simulink model "mobilesim1model"  (Simulink 6.6)
settings: Solver=ode3  StartTime=0.0  StopTime=100  FixedStep=dt  RelTol=1e-3
values from neighbouring files (symbols this model uses):
  D = 0.5    [mobile10demo.m]    (also in mobile2demo.m; mobilesim1demo.m; traje4demo.m = 1; vehi1demo.m)
  dt = 0.1    [mobile10demo.m]    (also in mobile2demo.m = 1; mobilesim1demo.m; traje1demo.m; traje2demo.m)
  theta0 = x0    [mobilesim1demo.m]
  xy = [x0(:),y0(:)]    [mobilesim1demo.m]
libraries: simulink x2
settings Model: Creator=root  LastModifiedBy=root
settings DebuggingCC: SignalResolutionControl=TryResolveAllWithWarning  MultiTaskDSMMsg=warning  MultiTaskCondExecSysMsg=none
settings RTWCC: IncludeERTFirstTime=on

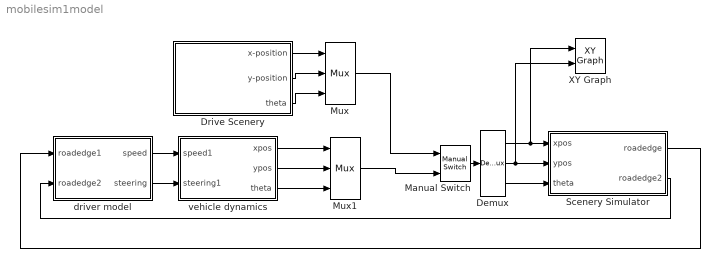
== system mobilesim1model ==
  Demux : Demux  Outputs=3
  Drive Scenery : Subsystem
  Manual Switch : simulink/Signal Routing/Manual Switch  SystemSampleTime=-1  sw=0  action=0  varsize=off
  Mux : Mux  Inputs=3
  Mux1 : Mux  Inputs=3
  Scenery Simulator : Subsystem
  XY Graph : simulink/Sinks/XY Graph  SystemSampleTime=-1  xmin=0  xmax=100  ymin=0  ymax=100  st=-1
  driver model : Subsystem
  vehicle dynamics : Subsystem
  wires:
  driver model/2(steering) -> vehicle dynamics/2(steering1)
  Scenery Simulator/2(roadedge2) -> driver model/2(roadedge2)
  Scenery Simulator/1(roadedge) -> driver model/1(roadedge1)
  driver model/1(speed) -> vehicle dynamics/1(speed1)
  Demux/1 -> Scenery Simulator/1(xpos), XY Graph/1
  Demux/2 -> Scenery Simulator/2(ypos), XY Graph/2
  Demux/3 -> Scenery Simulator/3(theta)
  Manual Switch/1 -> Demux/1
  vehicle dynamics/1(xpos) -> Mux1/1
  vehicle dynamics/2(ypos) -> Mux1/2
  vehicle dynamics/3(theta) -> Mux1/3
  Mux1/1 -> Manual Switch/2
  Mux/1 -> Manual Switch/1
  Drive Scenery/3(theta) -> Mux/3
  Drive Scenery/2(y-position) -> Mux/2
  Drive Scenery/1(x-position) -> Mux/1

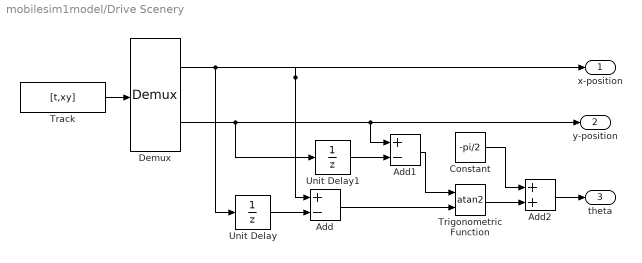
== system mobilesim1model/Drive Scenery ==
  Add : Sum  Inputs=+-  OutScaling=2^-10
  Add1 : Sum  Inputs=+-  OutScaling=2^-10
  Add2 : Sum  OutScaling=2^-10
  Constant : Constant  Value=-pi/2
  Demux : Demux  Outputs=2
  Track : FromWorkspace  VariableName=[t,xy]  SampleTime=dt
  Trigonometric Function : Trigonometry  Operator=atan2
  Unit Delay : UnitDelay  SampleTime=-1
  Unit Delay1 : UnitDelay  SampleTime=-1
  x-position : Outport
  y-position : Outport  Port=2
  theta : Outport  Port=3
  wires:
  Demux/2 -> Unit Delay1/1, y-position/1, Add1/1
  Demux/1 -> Unit Delay/1, Add/1, x-position/1
  Track/1 -> Demux/1
  Unit Delay/1 -> Add/2
  Add2/1 -> theta/1
  Constant/1 -> Add2/1
  Trigonometric Function/1 -> Add2/2
  Add/1 -> Trigonometric Function/2
  Add1/1 -> Trigonometric Function/1
  Unit Delay1/1 -> Add1/2

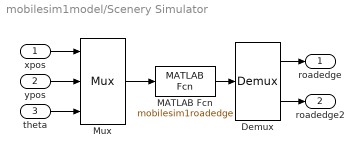
== system mobilesim1model/Scenery Simulator ==
  xpos : Inport
  ypos : Inport  Port=2
  theta : Inport  Port=3
  Demux : Demux  Outputs=2
  MATLAB Fcn : MATLABFcn  MATLABFcn=mobilesim1roadedge
  Mux : Mux  Inputs=3
  roadedge : Outport
  roadedge2 : Outport  Port=2
  wires:
  Mux/1 -> MATLAB Fcn/1
  MATLAB Fcn/1 -> Demux/1
  Demux/1 -> roadedge/1
  xpos/1 -> Mux/1
  ypos/1 -> Mux/2
  Demux/2 -> roadedge2/1
  theta/1 -> Mux/3

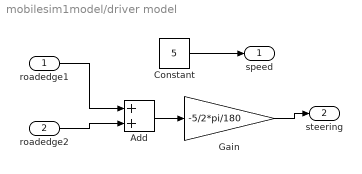
== system mobilesim1model/driver model ==
  roadedge1 : Inport
  roadedge2 : Inport  Port=2
  Add : Sum  OutScaling=2^-10
  Constant : Constant  Value=5
  Gain : Gain  Gain=-5/2*pi/180
  speed : Outport
  steering : Outport  Port=2
  wires:
  Constant/1 -> speed/1
  Gain/1 -> steering/1
  Add/1 -> Gain/1
  roadedge1/1 -> Add/1
  roadedge2/1 -> Add/2

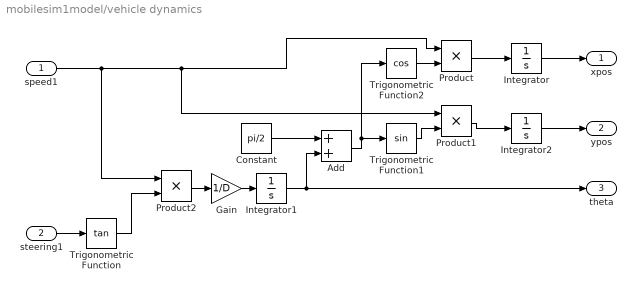
== system mobilesim1model/vehicle dynamics ==
  speed1 : Inport
  steering1 : Inport  Port=2
  Add : Sum  OutScaling=2^-10
  Constant : Constant  Value=pi/2
  Gain : Gain  Gain=1/D
  Integrator : Integrator  InitialCondition=xy(1,1)
  Integrator1 : Integrator  InitialCondition=theta0(1)
  Integrator2 : Integrator  InitialCondition=xy(1,2)
  Product : Product  RndMeth=Zero
  Product1 : Product  RndMeth=Zero
  Product2 : Product  RndMeth=Zero
  Trigonometric Function : Trigonometry  Operator=tan
  Trigonometric Function1 : Trigonometry
  Trigonometric Function2 : Trigonometry  Operator=cos
  xpos : Outport
  ypos : Outport  Port=2
  theta : Outport  Port=3
  wires:
  speed1/1 -> Product/1, Product1/1, Product2/1
  steering1/1 -> Trigonometric Function/1
  Gain/1 -> Integrator1/1
  Trigonometric Function1/1 -> Product1/2
  Product1/1 -> Integrator2/1
  Product/1 -> Integrator/1
  Integrator/1 -> xpos/1
  Integrator2/1 -> ypos/1
  Integrator1/1 -> theta/1, Add/2
  Trigonometric Function2/1 -> Product/2
  Trigonometric Function/1 -> Product2/2
  Product2/1 -> Gain/1
  Constant/1 -> Add/1
  Add/1 -> Trigonometric Function1/1, Trigonometric Function2/1
